simulink model "week3_proj3"  (R2021a)
settings: Solver=ode45  StartTime=0.0  StopTime=10.0  RelTol=1e-3
PreLoadFcn:
  | kp=100
  | ki=50
  | La=20
  | Ra=30
  | Kv=40
  | Bm=60
  | J=10
  | Kt=10
model workspace (MAT data in the model file):
  K = 50
undefined symbols (not defined in the file): sigbuilder_block
libraries: simulink_extras x1
settings Model: Creator=RASIKA MALGI  LastModifiedBy=RASIKA MALGI

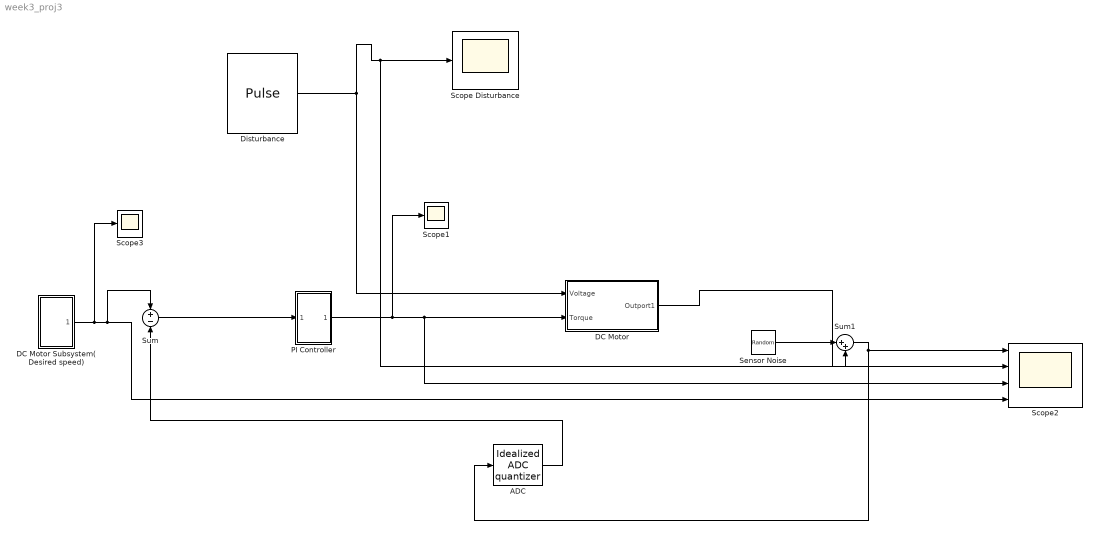
== system week3_proj3 ==
  ADC : simulink_extras/Additional Discrete/Idealized ADC quantizer  NumberOfConverterBits=12  Vmin=0  Vmax=5  OutputDataType=int16  OutputNegativeValues=off
  DC Motor : Subsystem
  DC Motor Subsystem(Desired speed) : Subsystem
  Disturbance : DiscretePulseGenerator  PulseType=Time based  Period=10  PulseWidth=5
  PI Controller : Subsystem
  Scope Disturbance : Scope
  Scope1 : Scope
  Scope2 : Scope  NumInputPorts=4
  Scope3 : Scope
  Sensor Noise : RandomNumber  SampleTime=0.1
  Sum : Sum  Inputs=+-
  Sum1 : Sum  Inputs=|++
  wires:
  ADC/1 -> Sum/2
  DC Motor/1(Outport1) -> Sum1/2
  Disturbance/1 -> DC Motor/1(Voltage), Scope2/2, Scope Disturbance/1
  Sum1/1 -> ADC/1, Scope2/1
  Sensor Noise/1 -> Sum1/1
  DC Motor Subsystem(Desired speed)/1(speed) -> Scope3/1, Scope2/4, Sum/1
  Sum/1 -> PI Controller/1(In1)
  PI Controller/1(Inport1) -> Scope1/1, Scope2/3, DC Motor/2(Torque)

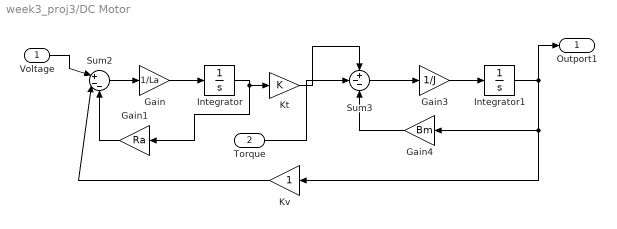
== system week3_proj3/DC Motor ==
  Voltage : Inport
  Torque : Inport  Port=2
  Gain : Gain  Gain=1/La
  Gain1 : Gain  Gain=Ra
  Gain3 : Gain  Gain=1/J
  Gain4 : Gain  Gain=Bm
  Integrator : Integrator
  Integrator1 : Integrator
  Kt : Gain  Gain=K
  Kv : Gain
  Sum2 : Sum  Inputs=|+--
  Sum3 : Sum  Inputs=+--
  Outport1 : Outport
  wires:
  Sum2/1 -> Gain/1
  Gain/1 -> Integrator/1
  Integrator/1 -> Gain1/1, Kt/1
  Gain3/1 -> Integrator1/1
  Integrator1/1 -> Outport1/1, Kv/1, Gain4/1
  Sum3/1 -> Gain3/1
  Gain4/1 -> Sum3/3
  Gain1/1 -> Sum2/3
  Voltage/1 -> Sum2/1
  Torque/1 -> Sum3/2
  Kt/1 -> Sum3/1
  Kv/1 -> Sum2/2

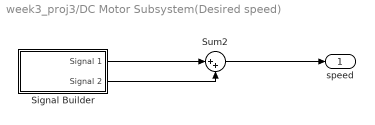
== system week3_proj3/DC Motor Subsystem(Desired speed) ==
  Signal Builder : Subsystem  Tag=STV Subsys  LoadFcn=sigbuilder_block('load');  StartFcn=sigbuilder_block('start');  StopFcn=sigbuilder_block('stop');  ClipboardFcn=sigbuilder_block('clipboard');  mask(Sigbuilder block){tuvar=[0:10]}
      mask help: Simulink:masks:SigbuilderBlock_MD
      mask init:
      | if ~strcmp(get_param(bdroot(gcbh),'SimulationStatus'),'stopped') tuvar = sigbuilder_block('maskInit'); end
      settings: CopyFcn=sigbuilder_block('copy');  DeleteFcn=sigbuilder_block('delete');  ModelCloseFcn=sigbuilder_block('modelClose');  PreSaveFcn=sigbuilder_block('preSave');  PauseFcn=sigbuilder_block('pause');  ContinueFcn=sigbuilder_block('continue');  NameChangeFcn=sigbuilder_block('namechange');  OpenFcn=sigbuilder_block('open',[437.6 199.2 550.4 400 ]);  CloseFcn=sigbuilder_block('close');
      mask Display: plot(0, 0, 100, 100,[2, 2, 32, 32, 2], [68, 8, 8, 68, 68],[32, 2], [38, 38], [32, 19, 2],[53, 60, 44], [32, 17, 17, 2],[16, 16, 31, 31]);txt = getActiveGroup(gcbh);text(2, 100, txt,'verticalAlignment', 'top');
  Sum2 : Sum  Inputs=|++
  speed : Outport
  wires:
  Signal Builder/2(Signal 2) -> Sum2/2
  Sum2/1 -> speed/1
  Signal Builder/1(Signal 1) -> Sum2/1

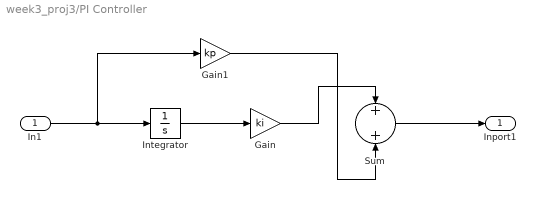
== system week3_proj3/PI Controller ==
  In1 : Inport
  Gain : Gain  Gain=ki
  Gain1 : Gain  Gain=kp
  Integrator : Integrator
  Sum : Sum
  Inport1 : Outport
  wires:
  Integrator/1 -> Gain/1
  Gain1/1 -> Sum/2
  In1/1 -> Gain1/1, Integrator/1
  Sum/1 -> Inport1/1
  Gain/1 -> Sum/1

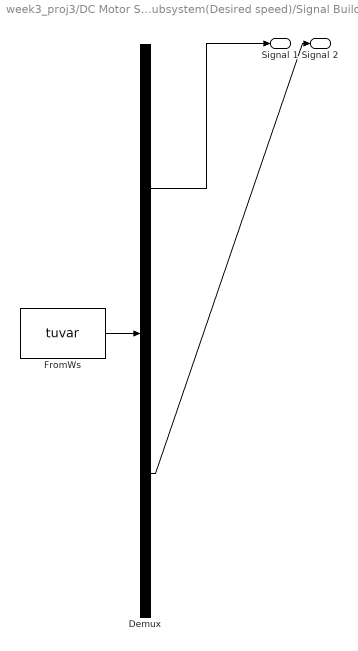
== system week3_proj3/DC Motor Subsystem(Desired speed)/Signal Builder ==
  Demux : Demux  Tag=STV Demux  Outputs=2
      settings: DisplayOption=none
  FromWs : FromWorkspace  Tag=STV FromWs  VariableName=tuvar
      SigBuilderData=|
      | common.afterFinalStr = 'Extrapolate'
      | common.sampleTime = 0
      | dataSet.timeRange = [0 10]
      | dataSet.name = 'Group 1'
      | sbobj.Groups.Name = 'Group 1'
      | sbobj.Groups.Signals(1).Name = 'Signal 1'
      | sbobj.Groups.Signals(1).XData = [0 5 5 10]
      | sbobj.Groups.Signals(1).YData = [0 0 1 1]
      | sbobj.Groups.Signals(2).Name = 'Signal 2'
      | sbobj.Groups.Signals(2).XData = [0 5 5 10]
      | sbobj.Groups.Signals(2).YData = [0 0 1 1]
  Signal 1 : Outport  Tag=STV Outport
  Signal 2 : Outport  Tag=STV Outport  Port=2
  wires:
  FromWs/1 -> Demux/1
  Demux/1 -> Signal 1/1
  Demux/2 -> Signal 2/1
